simulink model "v1"  (R2023a)
settings: Solver=VariableStepAuto  StartTime=0.0  StopTime=0.5  RelTol=1e-3
libraries: dspstat3 x3
settings Model: Creator=user  LastModifiedBy=user

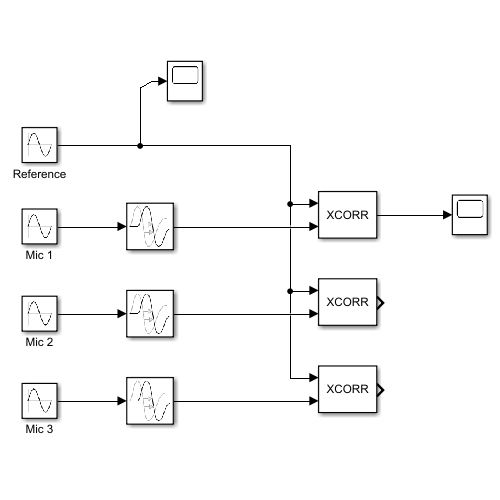
[thumbnail: Simulink's stored preview of the top-level diagram]
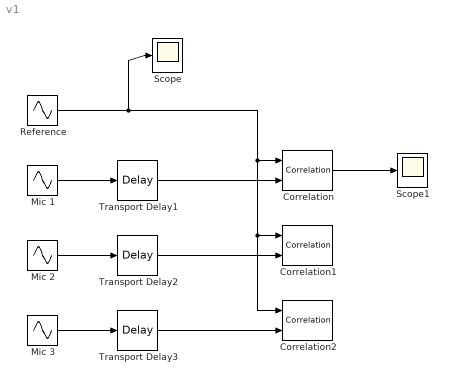
== system v1 ==
  Correlation : dspstat3/Correlation  domain=Time  roundingMode=Floor  overflowMode=off  outputDataTypeStr=Inherit: Same as accumulator  outputMin=[]  outputMax=[]  outputLastDataTypeStr=Inherit: Same as accumulator
  Correlation1 : dspstat3/Correlation  domain=Time  roundingMode=Floor  overflowMode=off  outputDataTypeStr=Inherit: Same as accumulator  outputMin=[]  outputMax=[]  outputLastDataTypeStr=Inherit: Same as accumulator
  Correlation2 : dspstat3/Correlation  domain=Time  roundingMode=Floor  overflowMode=off  outputDataTypeStr=Inherit: Same as accumulator  outputMin=[]  outputMax=[]  outputLastDataTypeStr=Inherit: Same as accumulator
  Mic 1 : Sin  Frequency=100  SampleTime=0
  Mic 2 : Sin  Frequency=100  SampleTime=0
  Mic 3 : Sin  Frequency=100  SampleTime=0
  Reference : Sin  Frequency=100  Samples=100000  SampleTime=0
  Scope : Scope
  Scope1 : Scope
  Transport Delay1 : TransportDelay  DelayTime=0.01
  Transport Delay2 : TransportDelay  DelayTime=0.01
  Transport Delay3 : TransportDelay  DelayTime=0.01
  wires:
  Mic 1/1 -> Transport Delay1/1
  Reference/1 -> Correlation2/1, Correlation1/1, Correlation/1, Scope/1
  Mic 2/1 -> Transport Delay2/1
  Mic 3/1 -> Transport Delay3/1
  Transport Delay1/1 -> Correlation/2
  Transport Delay3/1 -> Correlation2/2
  Transport Delay2/1 -> Correlation1/2
  Correlation/1 -> Scope1/1
